simulink model "mfsk_model_inclass"  (R2021b)
settings: Solver=VariableStepAuto  StartTime=0.0  StopTime=10.0  RelTol=1e-3
values from neighbouring files (symbols this model uses):
  Tb = 1/Rb    (= 0.0001)    [question2.m]
libraries: commutil2 x2, commdigbbndfm2 x2, commchan3 x1, commrandsrc3 x1, commsink2 x1
settings Model: Creator=enes_  LastModifiedBy=enes_

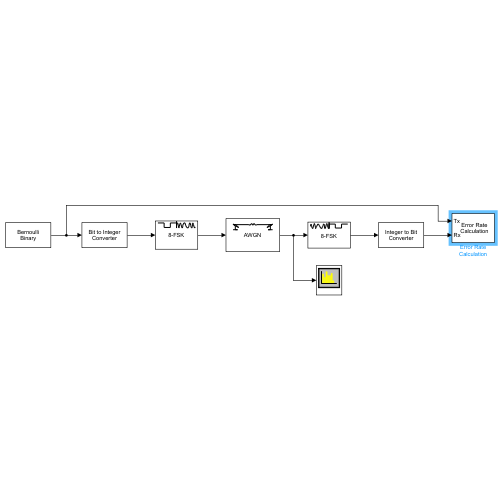
[thumbnail: Simulink's stored preview of the top-level diagram]
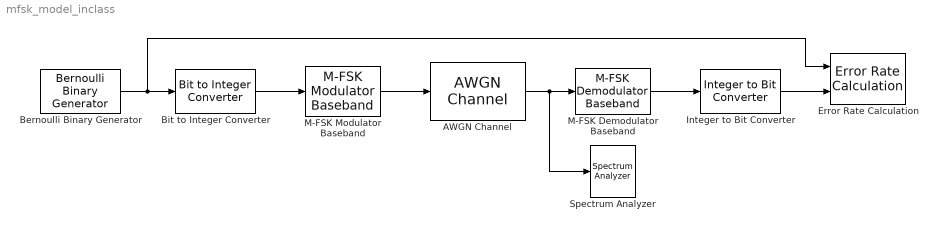
== system mfsk_model_inclass ==
  AWGN Channel : commchan3/AWGN Channel  InputProcessing=Columns as channels (frame based)  seed=67  noiseMode="Signal to noise ratio  (Eb/No)"  EbNodB=EbN0dB  EsNodB=10  SNRdB=10  bitsPerSym=k  Ps=1  Tsym=Ts  variance=1
  Bernoulli Binary Generator : commrandsrc3/Bernoulli Binary Generator  ProbabilityOfZero=0.5  SeedSource=Auto  Seed=0  SampleTime=Tb  SamplesPerFrame=3000  OutputDataType=double  SimulateUsing=Interpreted execution
  Bit to Integer Converter : commutil2/Bit to Integer Converter  nbits=k  bitOrder=MSB first  signedOutputValues=Unsigned  outDtype=Inherit via internal rule  outDtypeSigned=Inherit via internal rule
  Error Rate Calculation : commsink2/Error Rate Calculation  N=0  st_delay=0  cp_mode=Entire frame  subframe=[]  PMode=Workspace  WsName=ErrorVec  RsMode2=off  stop=off  numErr=100  maxBits=1e6
  Integer to Bit Converter : commutil2/Integer to Bit Converter  nbits=k  signedInputValues=Unsigned  bitOrder=MSB first  outDtype=Inherit via internal rule
  M-FSK Demodulator Baseband : commdigbbndfm2/M-FSK Demodulator Baseband  M=M  OutType=Integer  Dec=Gray  freqSep=Rs  numSamp=20  RateOptions=Enforce single-rate processing  outDataType=double
      settings: SourceProductBaseCode=CM
  M-FSK Modulator Baseband : commdigbbndfm2/M-FSK Modulator Baseband  M=M  InType=Integer  Enc=Gray  freqSep=Rs  phaseType=Continuous  numSamp=20  RateOptions=Enforce single-rate processing  outDataType=double
  Spectrum Analyzer : SpectrumAnalyzer
  wires:
  Bernoulli Binary Generator/1 -> Error Rate Calculation/1, Bit to Integer Converter/1
  Bit to Integer Converter/1 -> M-FSK Modulator Baseband/1
  M-FSK Modulator Baseband/1 -> AWGN Channel/1
  M-FSK Demodulator Baseband/1 -> Integer to Bit Converter/1
  Integer to Bit Converter/1 -> Error Rate Calculation/2
  AWGN Channel/1 -> Spectrum Analyzer/1, M-FSK Demodulator Baseband/1
